simulink model "my_robot"  (R2022b)
settings: Solver=VariableStepAuto  StartTime=0.0  StopTime=800  RelTol=1e-3
undefined symbols (not defined in the file or in its folder): DiscIntNeverNeededParam
libraries: simulink x2
settings Model: Creator=YawnFun  LastModifiedBy=YawnFun

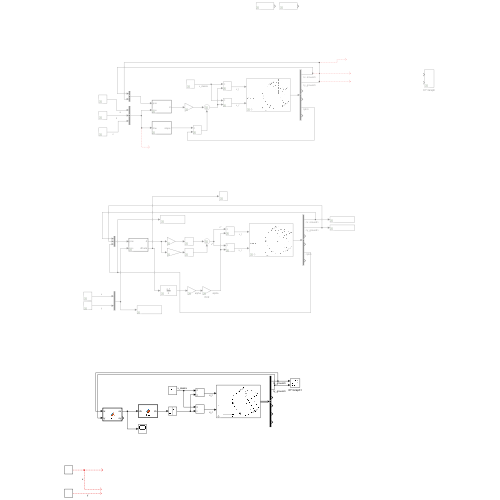
[thumbnail: Simulink's stored preview of the top-level diagram]
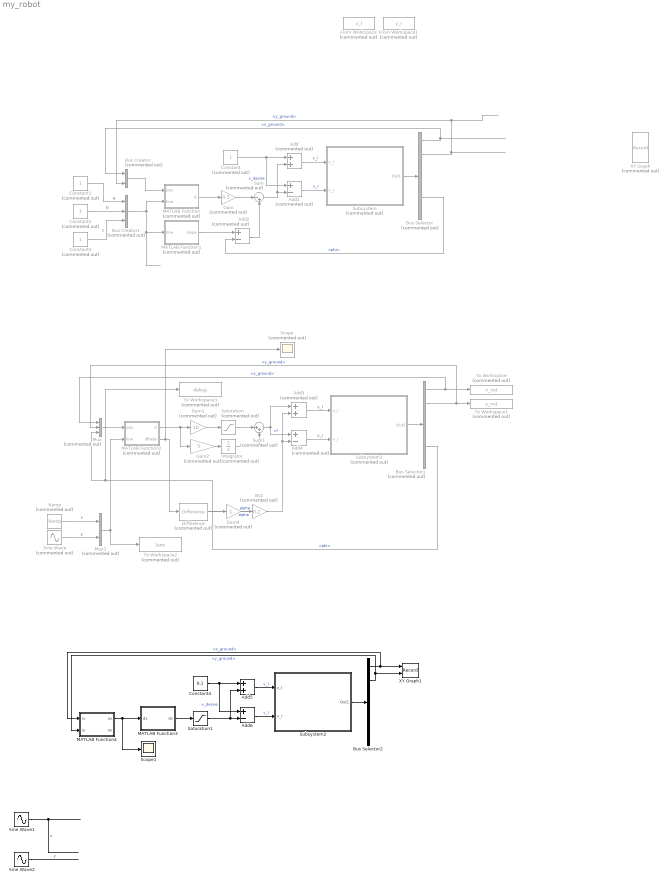
== system my_robot ==
  Add : Sum  Commented=on
  Add1 : Sum  Commented=on  Inputs=+-
  Add2 : Sum  Commented=on  Inputs=+-
  Add3 : Sum  Commented=on
  Add4 : Sum  Commented=on  Inputs=+-
  Add5 : Sum
  Add6 : Sum  Inputs=+-
  Bus Creator : BusCreator  Commented=on  Inputs=2
  Bus Creator1 : BusCreator  Commented=on  Inputs=3
  Bus Selector : BusSelector  Commented=on  OutputSignals=x_ground,y_ground,x_ground_dot,y_ground_dot,phi,phi_dot
  Bus Selector1 : BusSelector  Commented=on  OutputSignals=x_ground,y_ground,x_ground_dot,y_ground_dot,phi,phi_dot
  Bus Selector2 : BusSelector  OutputSignals=x_ground,y_ground,x_ground_dot,y_ground_dot,phi,phi_dot
  Constant{,1..3} (4 alike) : Constant  Commented=on
  Constant4 : Constant  Value=0.1
  Difference : simulink/Discrete/Difference  Commented=on  ICPrevInput=0.0  OutMin=[-10]  OutMax=[10]  OutDataType=fixdt(1, 16)  OutScaling=2^-10  DoSatur=off
  From Workspace : FromWorkspace  Commented=on  VariableName=v_l  SampleTime=0.01
  From Workspace1 : FromWorkspace  Commented=on  VariableName=v_r  SampleTime=0.01
  Gain : Gain  Commented=on  Gain=0.5
  Gain1 : Gain  Commented=on  Gain=10
  Gain2 : Gain  Commented=on  Gain=5
  Gain4 : Gain  Commented=on
  Integrator : Integrator  Commented=on  InitialCondition=0.0001  LimitOutput=on  UpperSaturationLimit=10  LowerSaturationLimit=-10
  MATLAB Function : MATLAB Function  Commented=on  TreatAsAtomicUnit=on
  MATLAB Function1 : MATLAB Function  Commented=on  TreatAsAtomicUnit=on
  MATLAB Function2 : MATLAB Function  Commented=on  TreatAsAtomicUnit=on
  MATLAB Function3 : MATLAB Function  TreatAsAtomicUnit=on
  MATLAB Function4 : MATLAB Function  TreatAsAtomicUnit=on
  Mux : Mux  Commented=on  Inputs=3
  Mux1 : Mux  Commented=on  Inputs=2
  Ramp : simulink/Sources/Ramp  Commented=on  slope=1  start=0  InitialOutput=0
  Saturation : Saturate  Commented=on  UpperLimit=10  LowerLimit=-10
  Saturation1 : Saturate  UpperLimit=0.2  LowerLimit=-0.2
  Scope : Scope  Commented=on
  Scope1 : Scope
  Sine Wave : Sin  Commented=on  Amplitude=0.1  Frequency=0.5*pi  SampleTime=0
  Sine Wave1 : Sin  Amplitude=4  Frequency=10  SampleTime=0
  Sine Wave2 : Sin  Frequency=10  Phase=pi/2  SampleTime=0
  Subsystem : Subsystem  Commented=on  mask{W=0.4, x_init=1, y_init=-4, phi_init=0, Ts=0.01}
      mask Display: image('C:\Users\YawnFun\Downloads\mulan_robot.png'); % Use "Edit Image" on toolstrip to change.
  Subsystem1 : Subsystem  Commented=on  mask{W=0.4, x_init=-1, y_init=-1, phi_init=1, Ts=0.01}
      mask Display: image('C:\Users\YawnFun\Downloads\mulan_robot.png'); % Use "Edit Image" on toolstrip to change.
  Subsystem2 : Subsystem  mask{W=0.4, x_init=-20, y_init=0, phi_init=0, Ts=0.01}
      mask Display: image('C:\Users\YawnFun\Downloads\mulan_robot.png'); % Use "Edit Image" on toolstrip to change.
  Sum : Sum  Commented=on  Inputs=|-+
  Sum1 : Sum  Commented=on  Inputs=|++
  To Workspace : ToWorkspace  Commented=on  VariableName=x_out  SaveFormat=Timeseries  SampleTime=-1
  To Workspace1 : ToWorkspace  Commented=on  VariableName=y_out  SaveFormat=Timeseries  SampleTime=-1
  To Workspace2 : ToWorkspace  Commented=on  VariableName=lane  SaveFormat=Timeseries  SampleTime=-1
  To Workspace3 : ToWorkspace  Commented=on  VariableName=debug  SaveFormat=Timeseries  SampleTime=-1
  W/2 : Gain  Commented=on  Gain=0.2
  XY Graph : Record  Commented=on  FileSettingsInternal="{\"entries\":[{\"content\":{\"excelSettings\":{\"content\":{},\"type\":\"Streamout.ExcelSettings\"}},\"type\":\"Streamout.FileSettingStorage\",\"uuid\":\"bdb3a574-d838-43e2-ae09-7d6c0c304725\"}],\"packageUris\":[\"http://schema.mathworks.com/mf0/streamout_blocks/R2020a\"],\"version\":\"1.0\"}"  Layout=[1 1]  SignalsInternal="{\"entries\":[{\"content\":{\"signals\":[]},\"type\":\"RecordBlkView.InputSignals\",\"uuid\":\"6165af37-410e-43dd-af1e-6381140384d4\"}],\"packageUris\":[\"http://schema.mathworks.com/mf0/streamout_blocks/R2020a\"],\"version\":\"1.0\"}"  VisualizationBindings="{\"xyplotplugin\":{\"info\":[{\"series\":[],\"subplotID\":1}]}}"  CompatibilityTag=XY
  XY Graph1 : Record  FileSettingsInternal="{\"entries\":[{\"content\":{\"excelSettings\":{\"content\":{},\"type\":\"Streamout.ExcelSettings\"}},\"type\":\"Streamout.FileSettingStorage\",\"uuid\":\"fdf883b4-203c-4155-91e6-a22af53581b9\"}],\"packageUris\":[\"http://schema.mathworks.com/mf0/streamout_blocks/R2020a\"],\"version\":\"1.0\"}"  Layout=[1 1]  SignalsInternal="{\"entries\":[{\"content\":{\"signals\":[{\"content\":{\"blockPath\":[\"my_robot/XY Graph1\"],\"channel\":[],\"dimensions\":[1],\"domain\":\"my_robot/XY Graph1\",\"lineColor\":\"#fe330a\",\"plots\":[1],\"port\":1,\"sid\":[\"\"],\"signalID\":248,\"signalName\":\"<x_ground>\"},\"type\":\"RecordBlkView.Signal\",\"uuid\":\"5379f1ab-1ebf-4c02-8e53-fe237d099e2e\"},{\"content\":{\"blockPath\":[\"my_robot/XY Graph1\"],\"channel\":[],\"dimensions\":[1],\"domain\":\"my_robot/XY Graph1\",\"lineColor\":\"#22b573\",\"plots\":[1],\"port\":2,\"sid\":[\"\"],\"signalID\":252,\"signalName\":\"<y_ground>\"},\"type\":\"RecordBlkView.Signal\",\"uuid\":\"a43f0f14-1c8a-4578-abd7-977e26e94073\"}]},\"type\":\"RecordBlkView.InputSignals\",\"uuid\":\"b3da2387-b802-44ae-953e-77b781d3acb7\"}],\"packageUris\":[\"http://schema.mathworks.com/mf0/streamout_blocks/R2020a\"],\"version\":\"1.0\"}"  VisualizationBindings="{\"xyplotplugin\":{\"info\":[{\"series\":[{\"bindingParametersList\":[{\"parameter\":\"X-Axis\",\"signalID\":248,\"signalName\":\"<x_ground>\"},{\"parameter\":\"Y-Axis\",\"signalID\":252,\"signalName\":\"<y_ground>\"}],\"seriesID\":4399}],\"subplotID\":1}]}}"  CompatibilityTag=XY
  wires:
  Subsystem/1(Out1) -> Bus Selector/1
  Bus Selector/1 -> Bus Creator/1  "<x_ground>"
  Bus Selector/2 -> Bus Creator/2  "<y_ground>"
  Bus Creator/1 -> MATLAB Function/1(pos)
  Constant/1 -> Add1/1, Add/1  "v_desire"
  Add/1 -> Subsystem/1(v_l)  "v_l"
  Add1/1 -> Subsystem/2(v_r)  "v_r"
  MATLAB Function/1(d) -> Gain/1
  Bus Selector/5 -> Add2/2  "<phi>"
  Add2/1 -> Sum/2
  Gain/1 -> Sum/1
  Bus Creator1/1 -> MATLAB Function/2(line), MATLAB Function1/1(line)
  Constant1/1 -> Bus Creator1/1  "a"
  Constant2/1 -> Bus Creator1/2  "b"
  Constant3/1 -> Bus Creator1/3  "c"
  MATLAB Function1/1(slope) -> Add2/1
  Sum/1 -> Add/2, Add1/2
  Bus Selector1/2 -> To Workspace1/1, Mux/2  "<y_ground>"
  Subsystem1/1(Out1) -> Bus Selector1/1
  Gain1/1 -> Saturation/1
  Bus Selector1/1 -> To Workspace/1, Mux/1  "<x_ground>"
  MATLAB Function2/2(dtheta) -> Scope/1, Difference/1
  Ramp/1 -> Mux1/1  "x"
  Add3/1 -> Subsystem1/1(v_l)  "v_l"
  Bus Selector1/5 -> Mux/3, To Workspace3/1  "<phi>"
  Add4/1 -> Subsystem1/2(v_r)  "v_r"
  Sine Wave/1 -> Mux1/2  "y"
  Mux1/1 -> To Workspace2/1, MATLAB Function2/2(line)
  Mux/1 -> MATLAB Function2/1(pos)
  MATLAB Function2/1(d) -> Gain2/1, Gain1/1
  Integrator/1 -> Sum1/2
  Sum1/1 -> Add3/1, Add4/1  "v*"
  Gain4/1 -> W/2/1  "alpha"
  Saturation/1 -> Sum1/1
  W/2/1 -> Add3/2, Add4/2  "alpha"
  Gain2/1 -> Integrator/1
  Difference/1 -> Gain4/1
  Add5/1 -> Subsystem2/1(v_l)  "v_l"
  Add6/1 -> Subsystem2/2(v_r)  "v_r"
  Subsystem2/1(Out1) -> Bus Selector2/1
  Constant4/1 -> Add6/1, Add5/1  "v_desire"
  Bus Selector2/1 -> XY Graph1/1, MATLAB Function4/1(ix)  "<x_ground>"
  Sine Wave2/1 -> ?  "y"
  Sine Wave1/1 -> ?  "x"
  Bus Selector2/2 -> XY Graph1/2, MATLAB Function4/2(iy)  "<y_ground>"
  MATLAB Function3/1(dv) -> Saturation1/1
  Saturation1/1 -> Add5/2, Add6/2
  MATLAB Function4/1(ox) -> Scope1/1, MATLAB Function3/1(dx)

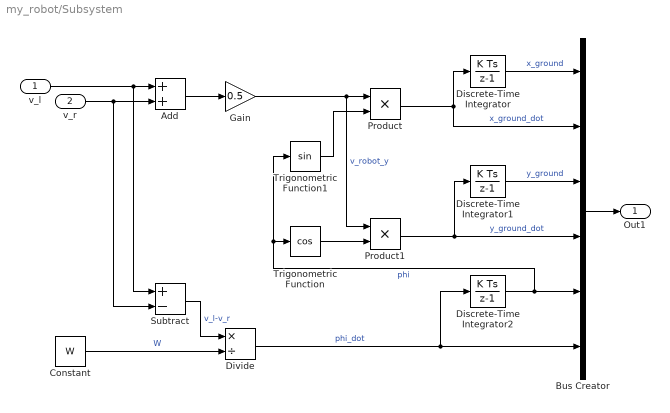
== system my_robot/Subsystem ==
  v_l : Inport
  v_r : Inport  Port=2
  Add : Sum
  Bus Creator : BusCreator  Inputs=6
  Constant : Constant  Value=W  VectorParams1D=off
  Discrete-Time Integrator : DiscreteIntegrator  InitialCondition=x_init  SampleTime=Ts  ICPrevOutput=DiscIntNeverNeededParam  ICPrevScaledInput=DiscIntNeverNeededParam
  Discrete-Time Integrator1 : DiscreteIntegrator  InitialCondition=y_init  SampleTime=Ts  ICPrevOutput=DiscIntNeverNeededParam  ICPrevScaledInput=DiscIntNeverNeededParam
  Discrete-Time Integrator2 : DiscreteIntegrator  InitialCondition=phi_init  SampleTime=Ts  ICPrevOutput=DiscIntNeverNeededParam  ICPrevScaledInput=DiscIntNeverNeededParam
  Divide : Product  Inputs=*/
  Gain : Gain  Gain=0.5
  Product : Product
  Product1 : Product
  Subtract : Sum  Inputs=+-
  Trigonometric Function : Trigonometry  Operator=cos
  Trigonometric Function1 : Trigonometry
  Out1 : Outport
  wires:
  Add/1 -> Gain/1
  Discrete-Time Integrator2/1 -> Trigonometric Function1/1, Trigonometric Function/1, Bus Creator/5  "phi"
  Product/1 -> Discrete-Time Integrator/1, Bus Creator/2  "x_ground_dot"
  Gain/1 -> Product/1, Product1/1  "v_robot_y"
  Bus Creator/1 -> Out1/1
  v_l/1 -> Subtract/1, Add/1
  v_r/1 -> Subtract/2, Add/2
  Discrete-Time Integrator/1 -> Bus Creator/1  "x_ground"
  Product1/1 -> Discrete-Time Integrator1/1, Bus Creator/4  "y_ground_dot"
  Discrete-Time Integrator1/1 -> Bus Creator/3  "y_ground"
  Divide/1 -> Discrete-Time Integrator2/1, Bus Creator/6  "phi_dot"
  Subtract/1 -> Divide/1  "v_l-v_r"
  Constant/1 -> Divide/2  "W"
  Trigonometric Function/1 -> Product1/2
  Trigonometric Function1/1 -> Product/2

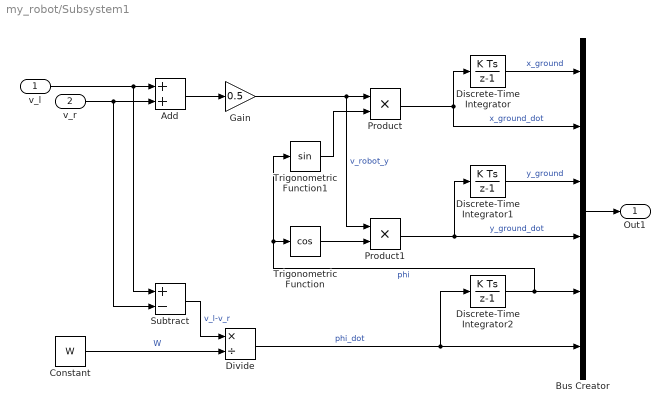
== system my_robot/Subsystem1 ==
  v_l : Inport
  v_r : Inport  Port=2
  Add : Sum
  Bus Creator : BusCreator  Inputs=6
  Constant : Constant  Value=W  VectorParams1D=off
  Discrete-Time Integrator : DiscreteIntegrator  InitialCondition=x_init  SampleTime=Ts  ICPrevOutput=DiscIntNeverNeededParam  ICPrevScaledInput=DiscIntNeverNeededParam
  Discrete-Time Integrator1 : DiscreteIntegrator  InitialCondition=y_init  SampleTime=Ts  ICPrevOutput=DiscIntNeverNeededParam  ICPrevScaledInput=DiscIntNeverNeededParam
  Discrete-Time Integrator2 : DiscreteIntegrator  InitialCondition=phi_init  SampleTime=Ts  ICPrevOutput=DiscIntNeverNeededParam  ICPrevScaledInput=DiscIntNeverNeededParam
  Divide : Product  Inputs=*/
  Gain : Gain  Gain=0.5
  Product : Product
  Product1 : Product
  Subtract : Sum  Inputs=+-
  Trigonometric Function : Trigonometry  Operator=cos
  Trigonometric Function1 : Trigonometry
  Out1 : Outport
  wires:
  Add/1 -> Gain/1
  Discrete-Time Integrator2/1 -> Trigonometric Function1/1, Trigonometric Function/1, Bus Creator/5  "phi"
  Product/1 -> Discrete-Time Integrator/1, Bus Creator/2  "x_ground_dot"
  Gain/1 -> Product/1, Product1/1  "v_robot_y"
  Bus Creator/1 -> Out1/1
  v_l/1 -> Subtract/1, Add/1
  v_r/1 -> Subtract/2, Add/2
  Discrete-Time Integrator/1 -> Bus Creator/1  "x_ground"
  Product1/1 -> Discrete-Time Integrator1/1, Bus Creator/4  "y_ground_dot"
  Discrete-Time Integrator1/1 -> Bus Creator/3  "y_ground"
  Divide/1 -> Discrete-Time Integrator2/1, Bus Creator/6  "phi_dot"
  Subtract/1 -> Divide/1  "v_l-v_r"
  Constant/1 -> Divide/2  "W"
  Trigonometric Function/1 -> Product1/2
  Trigonometric Function1/1 -> Product/2

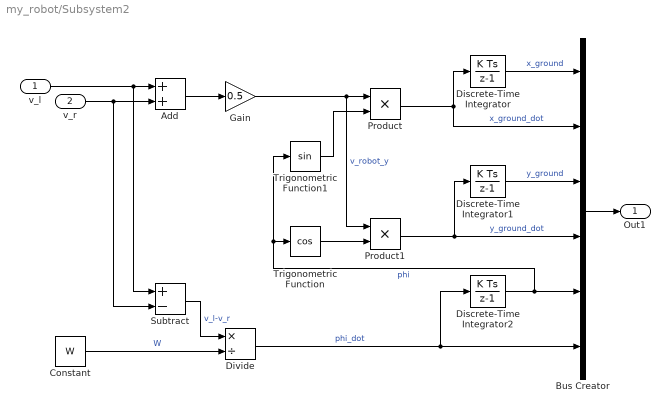
== system my_robot/Subsystem2 ==
  v_l : Inport
  v_r : Inport  Port=2
  Add : Sum
  Bus Creator : BusCreator  Inputs=6
  Constant : Constant  Value=W  VectorParams1D=off
  Discrete-Time Integrator : DiscreteIntegrator  InitialCondition=x_init  SampleTime=Ts  ICPrevOutput=DiscIntNeverNeededParam  ICPrevScaledInput=DiscIntNeverNeededParam
  Discrete-Time Integrator1 : DiscreteIntegrator  InitialCondition=y_init  SampleTime=Ts  ICPrevOutput=DiscIntNeverNeededParam  ICPrevScaledInput=DiscIntNeverNeededParam
  Discrete-Time Integrator2 : DiscreteIntegrator  InitialCondition=phi_init  SampleTime=Ts  ICPrevOutput=DiscIntNeverNeededParam  ICPrevScaledInput=DiscIntNeverNeededParam
  Divide : Product  Inputs=*/
  Gain : Gain  Gain=0.5
  Product : Product
  Product1 : Product
  Subtract : Sum  Inputs=+-
  Trigonometric Function : Trigonometry  Operator=cos
  Trigonometric Function1 : Trigonometry
  Out1 : Outport
  wires:
  Add/1 -> Gain/1
  Discrete-Time Integrator2/1 -> Trigonometric Function1/1, Trigonometric Function/1, Bus Creator/5  "phi"
  Product/1 -> Discrete-Time Integrator/1, Bus Creator/2  "x_ground_dot"
  Gain/1 -> Product/1, Product1/1  "v_robot_y"
  Bus Creator/1 -> Out1/1
  v_l/1 -> Subtract/1, Add/1
  v_r/1 -> Subtract/2, Add/2
  Discrete-Time Integrator/1 -> Bus Creator/1  "x_ground"
  Product1/1 -> Discrete-Time Integrator1/1, Bus Creator/4  "y_ground_dot"
  Discrete-Time Integrator1/1 -> Bus Creator/3  "y_ground"
  Divide/1 -> Discrete-Time Integrator2/1, Bus Creator/6  "phi_dot"
  Subtract/1 -> Divide/1  "v_l-v_r"
  Constant/1 -> Divide/2  "W"
  Trigonometric Function/1 -> Product1/2
  Trigonometric Function1/1 -> Product/2

== matlab function my_robot/MATLAB Function ==
  data: pos input; d output; line input
function d = fcn(pos,line)
x=pos(1);
y=pos(2);

a=line(1);
b=line(2);
c=line(3);

d=(a*x+b*y+c)/sqrt(a.^2+b.^2);

== matlab function my_robot/MATLAB Function2 ==
  data: pos input; d output; line input; dtheta output
function [d,dtheta] = fcn(pos,line)
x=pos(1);
y=pos(2);
phi=pos(3);

xx=line(1);
yy=line(2);


d=sqrt((xx-x)^2+(yy-y)^2)-0.1;

if xx>x
    dtheta=atan((xx-x)/(yy-y))-phi;
elseif xx<x
    dtheta=pi+atan((xx-x)/(yy-y))-phi;
else
    if yy>y
        dtheta=-phi;
    elseif yy<y
        dtheta=pi-phi;
    else
        dtheta=0;
    end
end

== matlab function my_robot/MATLAB Function3 ==
  data: dx input; dv output
function dv = fcn(dx)

dv=200./(1+exp(-(1/50)*dx))-100;

== matlab function my_robot/MATLAB Function4 ==
  data: ix input; iy input; ox output; oy output
function [ox,oy] = fcn(ix,iy)
% 椭圆路径x^2/400+y^2/100=1

if ix==0
    xx=0;
    if iy>0
        yy=1;
    else
        yy=0;
    end 
else
    xx=sqrt(400/(1+4*(iy/ix)^2));
    if ix<0
        xx=-xx;
    end
    yy=xx*iy/ix;
end
%disp(xx);
%disp(yy);

if (ix^2)/400+iy^2/100>=1
    ox=sqrt((ix-xx)^2+(iy-yy)^2);
else
    ox=-sqrt((ix-xx)^2+(iy-yy)^2);
end
oy=iy;

== matlab function my_robot/MATLAB Function1 ==
  data: line input; slope output
function slope = fcn(line)
slope=atan(-line(1)/line(2));
